simulink subsystem "high_fidelity_tilting_quadrotor"  (R2022b)
settings: Solver=VariableStepAuto  StartTime=0.0  StopTime=10.0  RelTol=1e-3
model mask{p0=[0 0 0], q0=[1 0 0 0], v0=[0 0 0], omega0=[0 0 0], alpha0=[0 0 0 0], d_alpha_0=[0 0 0 0], bar_w0=[0 0 0 0], m_b=2, beta=-pi/4 + pi/2*[0 2 1 3], I_b=eye(3), I_i=0.01*eye(3), c_direction=[ 1 1 -1 -1], k_m=1e-6, k_t=1e-5, p_mot=0.2*[cos(-pi/4+pi/2*[0 2 1 3]); sin(-pi/4+pi/2*[0 2 1 3]); 0 0 0 0], N=4}
  mask prompts: p0 "initial position [m]"; q0 "initial orientation [quaternion]"; v0 "initial linear velocity, world frame [m/s]"; omega0 "initial angular velocity, body frame [rad/s]"; alpha0 "initial tilting angles [rad]"; d_alpha_0 "initial tilting rate [rad/s]"; bar_w0 "initial propeller spinning rates"; m_b "quadrotor mass [Kg]"; beta "propeller mount vertical orientation"; I_b "main body inertia [Kg*m^2]"; I_i "propeller inertia [Kg*m^2]"; c_direction "propeller spinning direction (1:CCW, -1:CW)"; k_m "propeller drag constant [Nm/s^2]"; k_t "propeller thrust constant [N/s^2]"; p_mot "motor position"; N "number of propellers"
values from neighbouring files (symbols this model uses):
  beta = theta    [simple_high_fidelity_tilting_quadrotor_test_Data.m]
  c_direction = [1 1 -1 -1]    [simple_high_fidelity_tilting_quadrotor_test_Data.m]
  I_b = I_b - (stator.m+rotor.m+prop.m)*skew(p_mot(k,:))^2    [simple_high_fidelity_tilting_quadrotor_test_Data.m]
  I_i = I_prop+I_rotor    [simple_high_fidelity_tilting_quadrotor_test_Data.m]
  k_m = k_t * 0.01    [simple_high_fidelity_tilting_quadrotor_test_Data.m]
  k_t = prop.max_thrust / prop.w_max.^2    [simple_high_fidelity_tilting_quadrotor_test_Data.m]
  m_b = body.m + N*(stator.m+rotor.m+prop.m)    [simple_high_fidelity_tilting_quadrotor_test_Data.m]
  N = 4    [simple_high_fidelity_tilting_quadrotor_test_Data.m]
  p_mot = [ 0.2 -0.2 0 ... (first row only)    [simple_high_fidelity_tilting_quadrotor_test_Data.m]
settings Model: Creator=pozzan  LastModifiedBy=pozzan

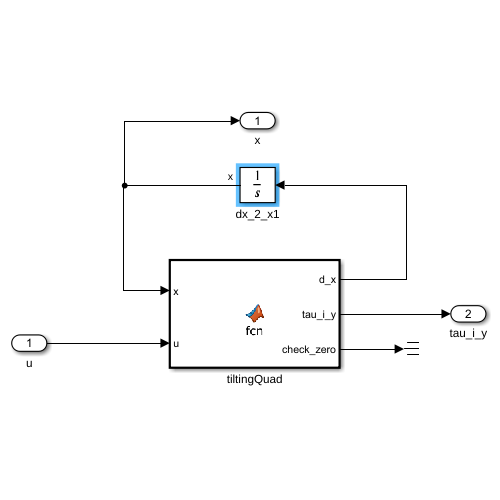
[thumbnail: Simulink's stored preview of the top-level diagram]
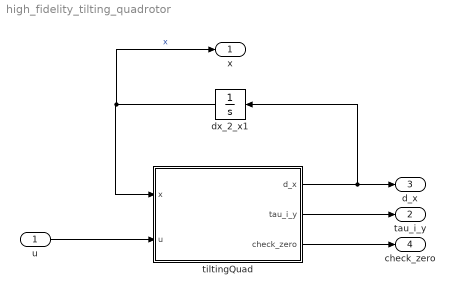
== system high_fidelity_tilting_quadrotor ==
  u : Inport
  dx_2_x1 : Integrator  InitialCondition=[p0(:); q0(:); v0(:); omega0(:); alpha0(:); d_alpha_0(:); bar_w0(:)]
  tiltingQuad : MATLAB Function  TreatAsAtomicUnit=on
  x : Outport
  tau_i_y : Outport  Port=2
  d_x : Outport  Port=3
  check_zero : Outport  Port=4
  wires:
  tiltingQuad/1(d_x) -> dx_2_x1/1, d_x/1
  dx_2_x1/1 -> x/1, tiltingQuad/1(x)  "x"
  tiltingQuad/3(check_zero) -> check_zero/1
  u/1 -> tiltingQuad/2(u)
  tiltingQuad/2(tau_i_y) -> tau_i_y/1

== matlab function high_fidelity_tilting_quadrotor/tiltingQuad ==
  data: x input; u input; d_x output; m_b parameter; beta parameter; I_b parameter; I_i parameter; c_direction parameter; k_m parameter; k_t parameter; p_mot parameter; tau_i_y output; N parameter; check_zero output
function [d_x, tau_i_y, check_zero] = fcn(x, u, m_b, beta, I_b, I_i, c_direction, k_m, k_t, p_mot, N)

% state x: [p q v omega alpha alpha_dot w_bar]
% input u: [tau_i_x tau_i_z]
% output:
%   dot_x
%   tau_i_y: contraint torques
%   check_zero
% parameters
%   m_b: drone mass [kg]
%   beta: propellers tilting plane yaw angle [rad]
%   I_b: main body inertia [Kg*m^2]
%   I_i: rotor+propeller inertia [Kg*m^2]
%   c_direction: propeller tourning direction (1:CCW, -1:CW)
%   k_m: propeller drag coefficient [Nm/s^2]
%   k_t: propeller torque coefficient [Nm/s^2]
%   p_mot: rotor position w.r.t. body

p_ind = 1:3;
q_ind = 4:7;
v_ind = 8:10;
omega_ind = 11:13;
alpha_ind = 14:14+N-1;
alpha_dot_ind = 14+N:14+2*N-1;
w_bar_ind = 14+2*N:14+3*N-1;

tau_i_x_ind = 1:N;
tau_i_z_ind = N+1:2*N;



% position of c.o.m. w.r.t. globa frame
p = x(p_ind);
% quaternion associated to B2W rotation
q = x(q_ind);
% linear velocity of c.o.m. expressed in world frame
v = x(v_ind);
% angular velocity expressed in body frame
omega = x(omega_ind);
% tilting angles
alpha = x(alpha_ind);
% tilting angle rates
alpha_dot = x(alpha_dot_ind);
% spinning rate
w_bar = x(w_bar_ind);

% tilting angle accelerations
tau_i_x = u(tau_i_x_ind);
% spinning rate accelerations
tau_i_z = u(tau_i_z_ind);

% output vector initialization
d_x = zeros(size(x));

check_zero = zeros(N,1);
alpha_ddot = zeros(size(alpha));
w_bar_dot = zeros(size(w_bar));

% body to world quaternion manipulation
eta = q(1);
epsilon = q(2:4);
epsilon_x = [
    0 -epsilon(3) epsilon(2)
    epsilon(3) 0 -epsilon(1)
    -epsilon(2) epsilon(1) 0
    ]; 
Rq = eye(3) + 2*eta*epsilon_x + 2*epsilon_x^2;          % rotation matrix, body to world
Mq = [eta, -epsilon'; epsilon, eta*eye(3)+epsilon_x];   % quaternion composition matrix
d_q = 1/2*Mq*[0;omega];                                 % quaternion derivative

coriol_b = cross(omega, I_b*omega);                      % coriolis componentes of the body

T_b = zeros(3,1);       % total body thrust
tau_b = zeros(3,1);     % total body torque (due to thrust)
b_tau_i = zeros(3,1);   % total internal torques (rotor-body) in body frame

%% constraint computation
% the constraint is in the form A_c*x_c+B_c=0
% x_c is the rotor y axis torque tau_i_y

A_c = zeros(N);
B_c = zeros(N,1);
c   = zeros(3,N);

for i=1:N
    B_R_i = axang2rotm([0 0 1 beta(i)])*axang2rotm([1 0 0 alpha(i)]);
    % thrust of i-th prop in **body** frame
    T_i = B_R_i* [0;0;c_direction(i)*k_t*w_bar(i)*abs(w_bar(i))];
    T_b = T_b + T_i;
    % body torque in body frame
    tau_b = tau_b + cross(p_mot(i,:)',T_i);
end

for i=1:N

    % rotor to body rotation matrix
    B_R_i = axang2rotm([0 0 1 beta(i)])*axang2rotm([1 0 0 alpha(i)]);
    % time derivative of rotor to body rotation matrix
    B_R_i_dot = B_R_i * ...
        [
        0       0       0
        0       0       -alpha_dot(i)
        0 alpha_dot(i)  0
        ];
    % angular velocity of the rotor in the rotor frame
    omega_i = B_R_i.' * omega + [alpha_dot(i); 0; w_bar(i)]; 
    coriol_i = cross(omega_i, I_i*omega_i);
    
    c_i_1 = I_i * B_R_i_dot*omega + coriol_i;
    
    c_i_2 = c_i_1 + I_i*B_R_i.'*(I_b\(tau_b-coriol_b));
    
    % tau_e_i, rotor drag torque = -k_m * w_bar * abs(w_bar)
    tau_ei = [0;0; -k_m*w_bar(i)*abs(w_bar(i))];
    
    c_i_3 = c_i_2 - tau_ei;

    c(:,i) = c_i_3;
    
    B_c(i) = [0 1 0]*(I_i\(c_i_3 - [tau_i_x(i); 0; tau_i_z(i)]));

    for j=1:N
        B_R_j = axang2rotm([0 0 1 beta(j)])*axang2rotm([1 0 0 alpha(j)]);
        i_I_b_j = B_R_j.'*I_b*B_R_i;
        A_c(i,j) = [0 1 0]*(i_I_b_j\[0;1;0]);

        B_c(i) = B_c(i) - [0 1 0]*(i_I_b_j\[tau_i_x(j); 0; tau_i_z(j)]);
    end
    A_c(i,i) = A_c(i,i) + [0 1 0]*(I_i\[0;1;0]);

end

tau_i_y = A_c\B_c;
    
% propeller torques composition in the rotor frames
tau_i = [
    tau_i_x.'
    tau_i_y.'
    tau_i_z.'
    ];

for i=1:N
    B_R_i = axang2rotm([0 0 1 beta(i)])*axang2rotm([1 0 0 alpha(i)]);
    b_tau_i = b_tau_i + B_R_i*tau_i(:,i);
end

d_v = [0;0;-9.81] + 1/m_b*Rq*T_b;
d_omega = I_b\(tau_b-coriol_b-b_tau_i);


for i=1:N
    B_R_i = axang2rotm([0 0 1 beta(i)])*axang2rotm([1 0 0 alpha(i)]);
    d_omega_rel = I_i\(tau_i(:,i) - c(:,i));
    for j = 1:N
        B_R_j = axang2rotm([0 0 1 beta(j)])*axang2rotm([1 0 0 alpha(j)]);
        i_I_b_j = B_R_j.'*I_b*B_R_i;
        d_omega_rel = d_omega_rel + i_I_b_j \ tau_i(:,j);
    end
    alpha_ddot(i)   = d_omega_rel(1);
    check_zero(i)   = d_omega_rel(2);
    w_bar_dot(i)    = d_omega_rel(3);
end



%% output filling

d_x(p_ind) = v;
d_x(q_ind) = d_q;
d_x(v_ind) = d_v;
d_x(omega_ind) = d_omega;
d_x(alpha_ind) = alpha_dot;
d_x(alpha_dot_ind) = alpha_ddot;
d_x(w_bar_ind) = w_bar_dot;
